simulink model "CDCDsimulink"  (R2024b)
settings: Solver=VariableStepAuto  StartTime=0.0  StopTime=0.01  RelTol=1e-3
InitFcn:
  | L=0.002;
  | R=10;
  | C=0.00001;
  | Uin=32;
  | DT=0.4;
settings Model: Creator=newju  LastModifiedBy=newju

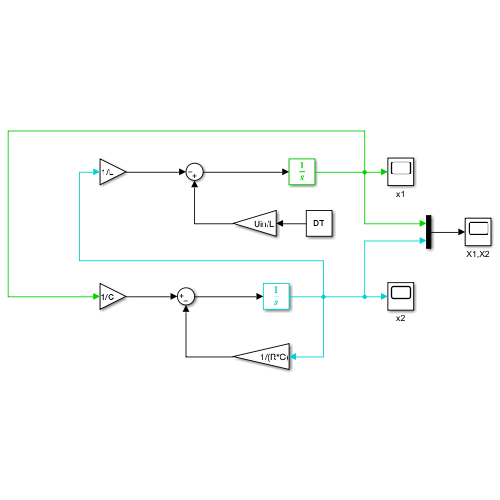
[thumbnail: Simulink's stored preview of the top-level diagram]
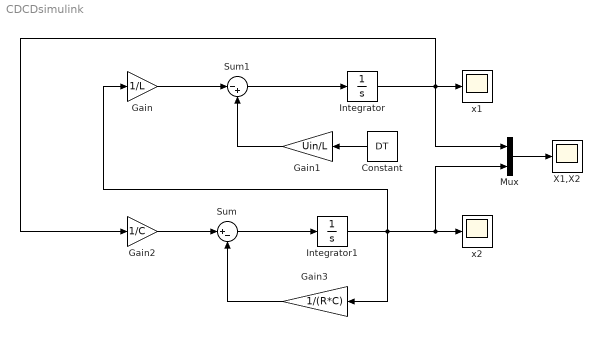
== system CDCDsimulink ==
  Constant : Constant  Value=DT
  Gain : Gain  Gain=1/L
  Gain1 : Gain  Gain=Uin/L
  Gain2 : Gain  Gain=1/C
  Gain3 : Gain  Gain=1/(R*C)
  Integrator : Integrator  InitialCondition=0.01
  Integrator1 : Integrator
  Mux : Mux  Inputs=2
  Sum : Sum  Inputs=|+-
  Sum1 : Sum  Inputs=|-+
  X1,X2 : Scope
  x1 : Scope
  x2 : Scope
  wires:
  Integrator/1 -> Mux/1, x1/1, Gain2/1
  Integrator1/1 -> Gain3/1, Gain/1, Mux/2, x2/1
  Mux/1 -> X1,X2/1
  Sum1/1 -> Integrator/1
  Sum/1 -> Integrator1/1
  Gain1/1 -> Sum1/2
  Gain/1 -> Sum1/1
  Constant/1 -> Gain1/1
  Gain2/1 -> Sum/1
  Gain3/1 -> Sum/2
